simulink model "Sim_Ex36_Quiz"  (R2017a)
settings: Solver=VariableStepAuto  StartTime=0.0  StopTime=Stop_Time  MaxStep=Ts  RelTol=1e-3
values from neighbouring files (symbols this model uses):
  Cdc = 3.3e-3    (= 0.0033)    [A_Ex36.m]
  Ls = 2e-3    (= 0.002)    [A_Ex36.m]
  Ls_Hat = 1.0*Ls    (= 0.002)    [A_Ex36.m]
  Pload = 0    [A_Ex36.m]
  Rs = 0.1    [A_Ex36.m]
  Time_Pload = 0.1    [A_Ex36.m]
  Time_Vdc_Ref = 0.1    [A_Ex36.m]
  Ts = 1/fs    (= 5e-05)    [A_Ex36.m]
  Tsw = 1/fsw    (= 0.0001)    [A_Ex36.m]
  Vdc_Init = 450    [A_Ex36.m]
  Vdc_Ref = Vdc_OP    (= 500)    [A_Ex36.m]
undefined symbols (not defined in the file or in its folder): CC, DiscIntNeverNeededParam, Grid, Mode, NF, PLL, VC
libraries: simulink x2
settings Model: SimulationMode=accelerator  Creator=Joonhee  LastModifiedBy=Joonhee
settings SolverCC: MaxConsecutiveMinStep=1000

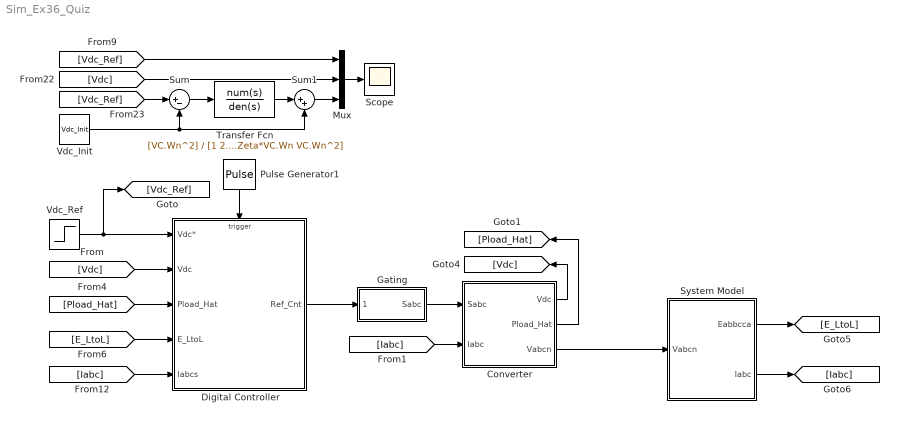
== system Sim_Ex36_Quiz ==
  Converter : Subsystem
  Digital Controller : Subsystem
  Gating : Subsystem
  Mux : Mux  Inputs=3
  Pulse Generator1 : DiscretePulseGenerator  PulseType=Time based  Period=Ts  PulseWidth=50
  Scope : Scope
  Sum : Sum  Inputs=|+-
  Sum1 : Sum  Inputs=|++
  System Model : Subsystem
  Transfer Fcn : TransferFcn  Numerator=[VC.Wn^2]  Denominator=[1 2*VC.Zeta*VC.Wn VC.Wn^2]
  Vdc_Init : Constant  Value=Vdc_Init
  Vdc_Ref : Step  Time=Time_Vdc_Ref  Before=Vdc_Init  After=Vdc_Ref  SampleTime=0
  wires:
  System Model/2(Iabc) -> [Iabc]
  [E_LtoL] -> Digital Controller/4(E_LtoL)
  Gating/1(Sabc) -> Converter/1(Sabc)
  System Model/1(Eabbcca) -> [E_LtoL]
  [Iabc] -> Converter/2(Iabc)
  [Iabc] -> Digital Controller/5(Iabcs)
  Pulse Generator1/1 -> Digital Controller/Trigger
  Converter/3(Vabcn) -> System Model/1(Vabcn)
  Digital Controller/1(Ref_Cnt) -> Gating/1(Ref_Cnt)
  Converter/1(Vdc) -> [Vdc]
  [Vdc] -> Digital Controller/2(Vdc)
  Vdc_Ref/1 -> [Vdc_Ref], Digital Controller/1(Vdc*)
  Converter/2(Pload_Hat) -> [Pload_Hat]
  [Pload_Hat] -> Digital Controller/3(Pload_Hat)
  [Vdc] -> Mux/2
  Sum1/1 -> Mux/3
  Mux/1 -> Scope/1
  Sum/1 -> Transfer Fcn/1
  [Vdc_Ref] -> Mux/1
  Vdc_Init/1 -> Sum1/2, Sum/2
  Transfer Fcn/1 -> Sum1/1
  [Vdc_Ref] -> Sum/1

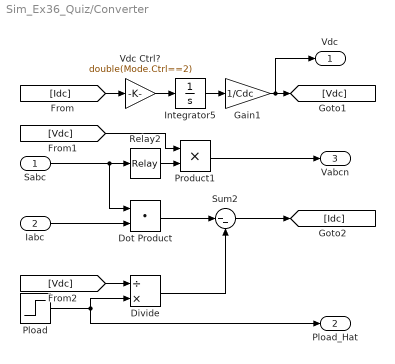
== system Sim_Ex36_Quiz/Converter ==
  Sabc : Inport
  Iabc : Inport  Port=2
  Divide : Product  Inputs=/*
  Dot Product : DotProduct  InputSameDT=on  OutDataTypeStr=Inherit: Inherit via internal rule
  Gain1 : Gain  Gain=1/Cdc
  Integrator5 : Integrator  InitialCondition=Cdc*Vdc_Init  LowerSaturationLimit=0
  Pload : Step  Time=Time_Pload  After=Pload  SampleTime=0
  Product1 : Product  RndMeth=Zero
  Relay2 : Relay  OnSwitchValue=0.5  OffSwitchValue=0.5  OnOutputValue=1/2  OffOutputValue=-1/2  OutDataTypeStr=double
  Sum2 : Sum  Inputs=|--
  Vdc Ctrl? : Gain  Gain=double(Mode.Ctrl==2)
  Vdc : Outport
  Pload_Hat : Outport  Port=2
  Vabcn : Outport  Port=3
  wires:
  [Vdc] -> Product1/1
  Sabc/1 -> Dot Product/1, Relay2/1
  Relay2/1 -> Product1/2
  Iabc/1 -> Dot Product/2
  Dot Product/1 -> Sum2/1
  Divide/1 -> Sum2/2
  Sum2/1 -> [Idc]
  Vdc Ctrl?/1 -> Integrator5/1
  Integrator5/1 -> Gain1/1
  Gain1/1 -> Vdc/1, [Vdc]
  [Idc] -> Vdc Ctrl?/1
  Product1/1 -> Vabcn/1
  [Vdc] -> Divide/1
  Pload/1 -> Pload_Hat/1, Divide/2

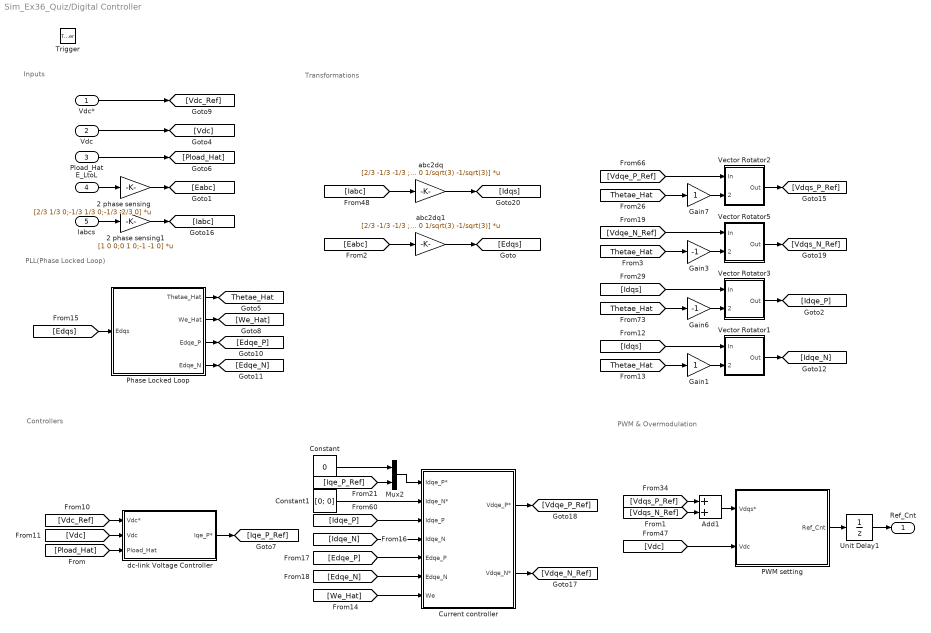
== system Sim_Ex36_Quiz/Digital Controller ==
  note: Controllers
  note: PLL(Phase Locked Loop)
  note: Inputs
  note: Transformations
  note: PWM & Overmodulation
  Vdc* : Inport
  Vdc : Inport  Port=2
  Pload_Hat : Inport  Port=3
  E_LtoL : Inport  Port=4
  Iabcs : Inport  Port=5
  Trigger : TriggerPort  VariantControl=Variant
  2 phase sensing : Gain  Gain=[2/3 1/3 0;-1/3 1/3 0;-1/3 -2/3 0]  Multiplication=Matrix(K*u)  SaturateOnIntegerOverflow=on  OutDataTypeStr=Inherit: Same as input  ParamDataTypeStr=Inherit: Same as input
  2 phase sensing1 : Gain  Gain=[1 0 0;0 1 0;-1 -1 0]  Multiplication=Matrix(K*u)  SaturateOnIntegerOverflow=on  OutDataTypeStr=Inherit: Same as input  ParamDataTypeStr=Inherit: Same as input
  Add1 : Sum
  Constant : Constant  Value=0
  Constant1 : Constant  Value=[0; 0]
  Current controller : Subsystem
  Gain1 : Gain
  Gain3 : Gain  Gain=-1
  Gain6 : Gain  Gain=-1
  Gain7 : Gain
  Mux2 : Mux  Inputs=2
  PWM setting : Subsystem
  Phase Locked Loop : Subsystem
  Unit Delay1 : UnitDelay  SampleTime=-1
  Vector Rotator1 : Subsystem
  Vector Rotator2 : Subsystem
  Vector Rotator3 : Subsystem
  Vector Rotator5 : Subsystem
  abc2dq : Gain  Gain=[2/3 -1/3 -1/3 ; 0 1/sqrt(3) -1/sqrt(3)]  Multiplication=Matrix(K*u)  SaturateOnIntegerOverflow=on  OutDataTypeStr=Inherit: Same as input  ParamDataTypeStr=Inherit: Same as input
  abc2dq1 : Gain  Gain=[2/3 -1/3 -1/3 ; 0 1/sqrt(3) -1/sqrt(3)]  Multiplication=Matrix(K*u)  SaturateOnIntegerOverflow=on  OutDataTypeStr=Inherit: Same as input  ParamDataTypeStr=Inherit: Same as input
  dc-link Voltage Controller : Subsystem
  Ref_Cnt : Outport  InitialOutput=[0]
  tag scope: Thetae_Hat=global
  wires:
  [Idqe_P] -> Current controller/3(Idqe_P)
  abc2dq/1 -> [Idqs]
  [Iabc] -> abc2dq/1
  [We_Hat] -> Current controller/7(We)
  Unit Delay1/1 -> Ref_Cnt/1
  [Thetae_Hat] -> Gain7/1
  Gain7/1 -> Vector Rotator2/2(Theta)
  [Vdqe_P_Ref] -> Vector Rotator2/1(In)
  Vector Rotator2/1(Out) -> [Vdqs_P_Ref]
  Gain6/1 -> Vector Rotator3/2(Theta)
  [Idqs] -> Vector Rotator3/1(In)
  Vector Rotator3/1(Out) -> [Idqe_P]
  [Thetae_Hat] -> Gain6/1
  Iabcs/1 -> 2 phase sensing1/1
  2 phase sensing1/1 -> [Iabc]
  [Edqs] -> Phase Locked Loop/1(Edqs)
  2 phase sensing/1 -> [Eabc]
  E_LtoL/1 -> 2 phase sensing/1
  [Eabc] -> abc2dq1/1
  abc2dq1/1 -> [Edqs]
  Phase Locked Loop/2(We_Hat) -> [We_Hat]
  [Edqe_P] -> Current controller/5(Edqe_P)
  [Edqe_N] -> Current controller/6(Edqe_N)
  [Thetae_Hat] -> Gain1/1
  Vector Rotator1/1(Out) -> [Idqe_N]
  Gain1/1 -> Vector Rotator1/2(Theta)
  [Idqs] -> Vector Rotator1/1(In)
  Current controller/2(Vdqe_N*) -> [Vdqe_N_Ref]
  [Idqe_N] -> Current controller/4(Idqe_N)
  Vector Rotator5/1(Out) -> [Vdqs_N_Ref]
  [Vdqe_N_Ref] -> Vector Rotator5/1(In)
  Gain3/1 -> Vector Rotator5/2(Theta)
  [Thetae_Hat] -> Gain3/1
  Phase Locked Loop/3(Edqe_P) -> [Edqe_P]
  Phase Locked Loop/4(Edqe_N) -> [Edqe_N]
  Phase Locked Loop/1(Thetae_Hat) -> [Thetae_Hat]
  Current controller/1(Vdqe_P*) -> [Vdqe_P_Ref]
  Vdc/1 -> [Vdc]
  dc-link Voltage Controller/1(Iqe_P*) -> [Iqe_P_Ref]
  [Vdc] -> dc-link Voltage Controller/2(Vdc)
  [Vdc_Ref] -> dc-link Voltage Controller/1(Vdc*)
  Vdc*/1 -> [Vdc_Ref]
  [Iqe_P_Ref] -> Mux2/2
  Mux2/1 -> Current controller/1(Idqe_P*)
  Constant/1 -> Mux2/1
  Pload_Hat/1 -> [Pload_Hat]
  [Pload_Hat] -> dc-link Voltage Controller/3(Pload_Hat)
  [Vdc] -> PWM setting/2(Vdc)
  [Vdqs_P_Ref] -> Add1/1
  [Vdqs_N_Ref] -> Add1/2
  PWM setting/1(Ref_Cnt) -> Unit Delay1/1
  Add1/1 -> PWM setting/1(Vdqs*)
  Constant1/1 -> Current controller/2(Idqe_N*)

== system Sim_Ex36_Quiz/Gating ==
  Ref_Cnt : Inport
  Add3 : Sum  Inputs=+-
  Relay3 : Relay  OnSwitchValue=10*eps  OffSwitchValue=-10*eps  OutDataTypeStr=double
  Repeating Sequence1 : simulink/Sources/Repeating Sequence  rep_seq_t=[0 Tsw/2 Tsw]  rep_seq_y=[0 1 0]
  Sabc : Outport
  wires:
  Add3/1 -> Relay3/1
  Relay3/1 -> Sabc/1
  Repeating Sequence1/1 -> Add3/2
  Ref_Cnt/1 -> Add3/1

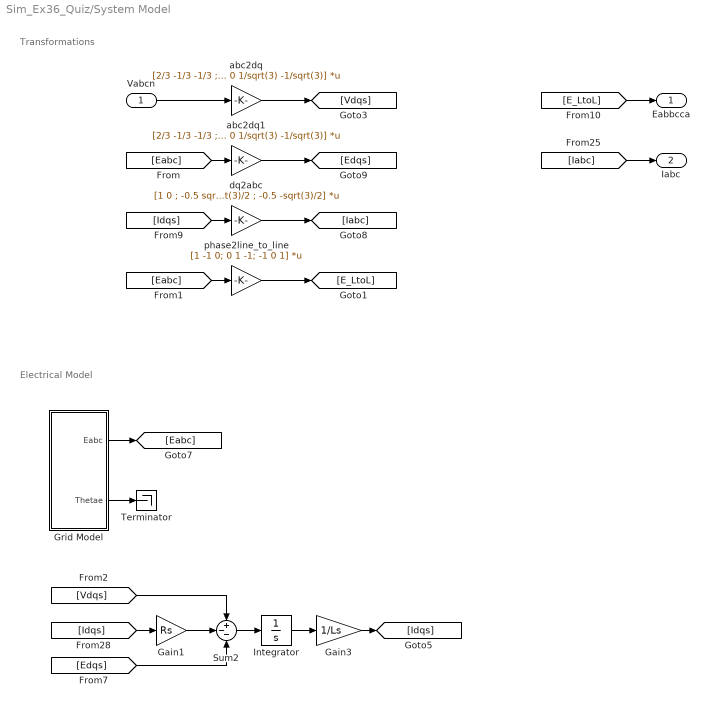
== system Sim_Ex36_Quiz/System Model ==
  note: Electrical Model
  note: Transformations
  Vabcn : Inport
  Gain1 : Gain  Gain=Rs
  Gain3 : Gain  Gain=1/Ls
  Grid Model : Subsystem
  Integrator : Integrator
  Sum2 : Sum  Inputs=+--
  Terminator : Terminator
  abc2dq : Gain  Gain=[2/3 -1/3 -1/3 ; 0 1/sqrt(3) -1/sqrt(3)]  Multiplication=Matrix(K*u)  SaturateOnIntegerOverflow=on  OutDataTypeStr=Inherit: Same as input  ParamDataTypeStr=Inherit: Same as input
  abc2dq1 : Gain  Gain=[2/3 -1/3 -1/3 ; 0 1/sqrt(3) -1/sqrt(3)]  Multiplication=Matrix(K*u)  SaturateOnIntegerOverflow=on  OutDataTypeStr=Inherit: Same as input  ParamDataTypeStr=Inherit: Same as input
  dq2abc : Gain  Gain=[1 0 ; -0.5 sqrt(3)/2 ; -0.5 -sqrt(3)/2]  Multiplication=Matrix(K*u)
  phase2line_to_line : Gain  Gain=[1 -1 0; 0 1 -1; -1 0 1]  Multiplication=Matrix(K*u)
  Eabbcca : Outport
  Iabc : Outport  Port=2
  wires:
  [Idqs] -> Gain1/1
  Vabcn/1 -> abc2dq/1
  [Idqs] -> dq2abc/1
  dq2abc/1 -> [Iabc]
  [Iabc] -> Iabc/1
  [Eabc] -> abc2dq1/1
  abc2dq1/1 -> [Edqs]
  Integrator/1 -> Gain3/1
  Gain3/1 -> [Idqs]
  Sum2/1 -> Integrator/1
  [E_LtoL] -> Eabbcca/1
  abc2dq/1 -> [Vdqs]
  [Vdqs] -> Sum2/1
  [Eabc] -> phase2line_to_line/1
  phase2line_to_line/1 -> [E_LtoL]
  Gain1/1 -> Sum2/2
  [Edqs] -> Sum2/3
  Grid Model/2(Thetae) -> Terminator/1
  Grid Model/1(Eabc) -> [Eabc]

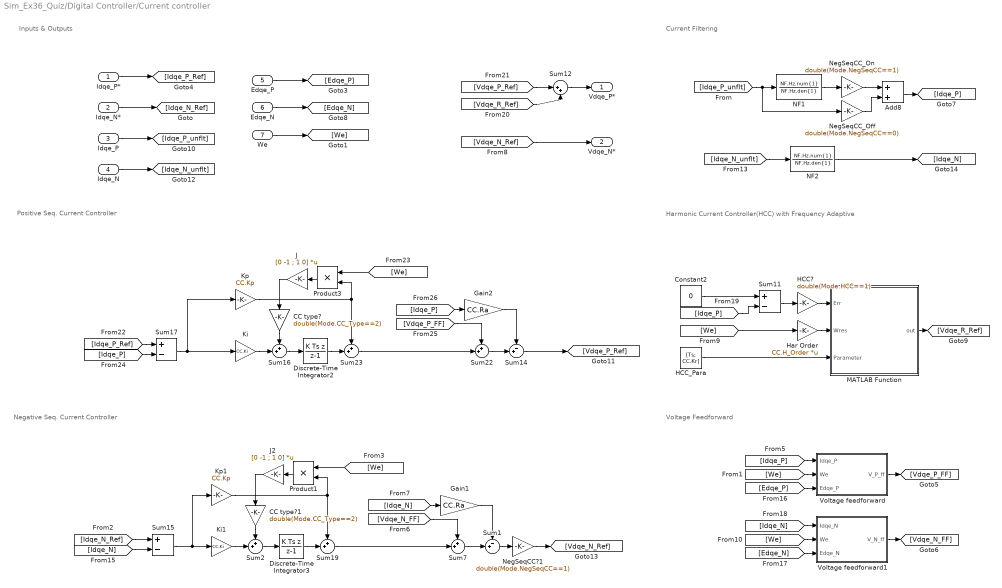
== system Sim_Ex36_Quiz/Digital Controller/Current controller ==
  note: Positive Seq. Current Controller
  note: Negative Seq. Current Controller
  note: Inputs & Outputs
  note: Voltage Feedforward
  note: Harmonic Current Controller(HCC)
      | with Frequency Adaptive
  note: Current Filtering
  Idqe_P* : Inport
  Idqe_N* : Inport  Port=2
  Idqe_P : Inport  Port=3
  Idqe_N : Inport  Port=4
  Edqe_P : Inport  Port=5
  Edqe_N : Inport  Port=6
  We : Inport  Port=7
  Add8 : Sum
  CC type? : Gain  Gain=double(Mode.CC_Type==2)
  CC type?1 : Gain  Gain=double(Mode.CC_Type==2)
  Constant2 : Constant  Value=0
  Discrete-Time Integrator2 : DiscreteIntegrator  IntegratorMethod=Integration: Backward Euler  SampleTime=-1  ICPrevOutput=DiscIntNeverNeededParam  ICPrevScaledInput=DiscIntNeverNeededParam
  Discrete-Time Integrator3 : DiscreteIntegrator  IntegratorMethod=Integration: Backward Euler  SampleTime=-1  ICPrevOutput=DiscIntNeverNeededParam  ICPrevScaledInput=DiscIntNeverNeededParam
  Gain1 : Gain  Gain=CC.Ra
  Gain2 : Gain  Gain=CC.Ra
  HCC? : Gain  Gain=double(Mode.HCC==1)
  HCC_Para : Constant  Value=[Ts; CC.Kr]
  Har Order : Gain  Gain=CC.H_Order  Multiplication=Matrix(K*u)
  J : Gain  Gain=[0 -1 ; 1 0]  Multiplication=Matrix(K*u)
  J2 : Gain  Gain=[0 -1 ; 1 0]  Multiplication=Matrix(K*u)
  Ki : Gain  Gain=CC.Ki  SaturateOnIntegerOverflow=on  OutDataTypeStr=Inherit: Same as input  ParamDataTypeStr=Inherit: Same as input
  Ki1 : Gain  Gain=CC.Ki  SaturateOnIntegerOverflow=on  OutDataTypeStr=Inherit: Same as input  ParamDataTypeStr=Inherit: Same as input
  Kp : Gain  Gain=CC.Kp  SaturateOnIntegerOverflow=on  OutDataTypeStr=Inherit: Same as input  ParamDataTypeStr=Inherit: Same as input
  Kp1 : Gain  Gain=CC.Kp  SaturateOnIntegerOverflow=on  OutDataTypeStr=Inherit: Same as input  ParamDataTypeStr=Inherit: Same as input
  MATLAB Function : MATLAB Function  TreatAsAtomicUnit=on
  NF1 : DiscreteFilter  Numerator=NF.Hz.num{1}  Denominator=NF.Hz.den{1}
  NF2 : DiscreteFilter  Numerator=NF.Hz.num{1}  Denominator=NF.Hz.den{1}
  NegSeqCC?1 : Gain  Gain=double(Mode.NegSeqCC==1)
  NegSeqCC_Off : Gain  Gain=double(Mode.NegSeqCC==0)
  NegSeqCC_On : Gain  Gain=double(Mode.NegSeqCC==1)
  Product1 : Product  RndMeth=Zero
  Product3 : Product  RndMeth=Zero
  Sum1 : Sum  Inputs=-+|
  Sum11 : Sum  Inputs=+-
  Sum12 : Sum  Inputs=|++
  Sum14 : Sum  Inputs=-+|
  Sum15 : Sum  Inputs=+-
  Sum{2,7,16,19,22..23} (6 alike) : Sum  Inputs=++|
  Sum17 : Sum  Inputs=+-
  Voltage feedforward : Subsystem
  Voltage feedforward1 : Subsystem
  Vdqe_P* : Outport
  Vdqe_N* : Outport  Port=2
  wires:
  Sum11/1 -> HCC?/1
  HCC_Para/1 -> MATLAB Function/3(Parameter)
  HCC?/1 -> MATLAB Function/1(Err)
  MATLAB Function/1(out) -> [Vdqe_R_Ref]
  Har Order/1 -> MATLAB Function/2(Wres)
  [Idqe_P] -> Sum11/2
  Constant2/1 -> Sum11/1
  [We] -> Har Order/1
  Voltage feedforward/1(V_P_ff) -> [Vdqe_P_FF]
  [Idqe_P] -> Voltage feedforward/1(Idqe_P)
  [Edqe_P] -> Voltage feedforward/3(Edqe_P)
  [We] -> Voltage feedforward1/2(We)
  [Edqe_N] -> Voltage feedforward1/3(Edqe_N)
  Voltage feedforward1/1(V_N_ff) -> [Vdqe_N_FF]
  [Idqe_N] -> Voltage feedforward1/1(Idqe_N)
  [We] -> Voltage feedforward/2(We)
  Discrete-Time Integrator2/1 -> Sum23/2
  Kp/1 -> Product3/2, Sum23/1
  Sum16/1 -> Discrete-Time Integrator2/1
  Sum14/1 -> [Vdqe_P_Ref]
  Gain2/1 -> Sum14/1
  Sum17/1 -> Ki/1, Kp/1
  [Idqe_P] -> Sum17/2
  CC type?/1 -> Sum16/1
  [Vdqe_P_FF] -> Sum22/1
  Ki/1 -> Sum16/2
  J/1 -> CC type?/1
  Sum23/1 -> Sum22/2
  [Idqe_P] -> Gain2/1
  [We] -> Product3/1
  [Idqe_P_Ref] -> Sum17/1
  Sum22/1 -> Sum14/2
  Product3/1 -> J/1
  Discrete-Time Integrator3/1 -> Sum19/2
  Sum19/1 -> Sum7/2
  [Idqe_N_Ref] -> Sum15/1
  Kp1/1 -> Product1/2, Sum19/1
  CC type?1/1 -> Sum2/1
  [Idqe_N] -> Sum15/2
  NegSeqCC?1/1 -> [Vdqe_N_Ref]
  Sum7/1 -> Sum1/2
  Sum1/1 -> NegSeqCC?1/1
  Sum15/1 -> Ki1/1, Kp1/1
  [Idqe_N] -> Gain1/1
  [We] -> Product1/1
  Ki1/1 -> Sum2/2
  [Vdqe_N_FF] -> Sum7/1
  Gain1/1 -> Sum1/1
  Sum2/1 -> Discrete-Time Integrator3/1
  Product1/1 -> J2/1
  J2/1 -> CC type?1/1
  Idqe_N*/1 -> [Idqe_N_Ref]
  [Vdqe_R_Ref] -> Sum12/2
  Idqe_P/1 -> [Idqe_P_unflt]
  Sum12/1 -> Vdqe_P*/1
  [Vdqe_P_Ref] -> Sum12/1
  Edqe_P/1 -> [Edqe_P]
  [Vdqe_N_Ref] -> Vdqe_N*/1
  Edqe_N/1 -> [Edqe_N]
  Idqe_N/1 -> [Idqe_N_unflt]
  Idqe_P*/1 -> [Idqe_P_Ref]
  We/1 -> [We]
  [Idqe_N_unflt] -> NF2/1
  NF2/1 -> [Idqe_N]
  NegSeqCC_On/1 -> Add8/1
  [Idqe_P_unflt] -> NegSeqCC_Off/1, NF1/1
  Add8/1 -> [Idqe_P]
  NF1/1 -> NegSeqCC_On/1
  NegSeqCC_Off/1 -> Add8/2

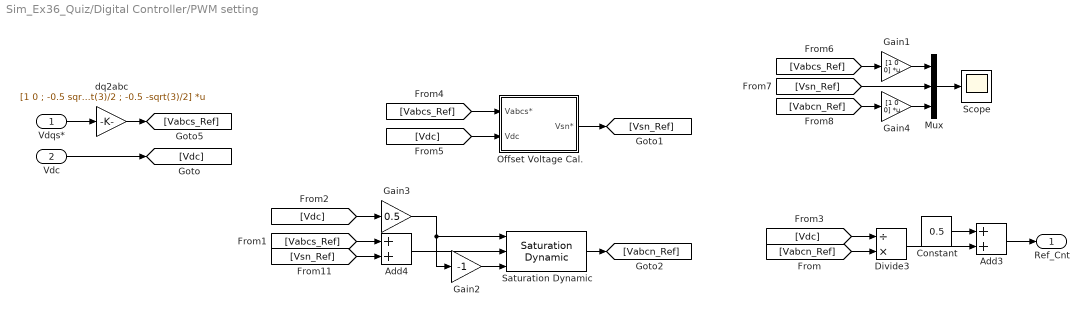
== system Sim_Ex36_Quiz/Digital Controller/PWM setting ==
  Vdqs* : Inport
  Vdc : Inport  Port=2
  Add3 : Sum
  Add4 : Sum
  Constant : Constant  Value=0.5
  Divide3 : Product  Inputs=/*
  Gain1 : Gain  Gain=[1 0 0]  Multiplication=Matrix(K*u)
  Gain2 : Gain  Gain=-1
  Gain3 : Gain  Gain=0.5
  Gain4 : Gain  Gain=[1 0 0]  Multiplication=Matrix(K*u)
  Mux : Mux  Inputs=3
  Offset Voltage Cal. : Subsystem
  Saturation Dynamic : simulink/Discontinuities/Saturation Dynamic  OutMin=[]  OutMax=[]  OutDataTypeStr=Inherit: Same as second input  OutDataType=fixdt(1, 16)  OutScaling=2^-10  DoSatur=off
  Scope : Scope
  dq2abc : Gain  Gain=[1 0 ; -0.5 sqrt(3)/2 ; -0.5 -sqrt(3)/2]  Multiplication=Matrix(K*u)
  Ref_Cnt : Outport
  wires:
  [Vdc] -> Divide3/1
  Divide3/1 -> Add3/2
  Add3/1 -> Ref_Cnt/1
  Constant/1 -> Add3/1
  Vdqs*/1 -> dq2abc/1
  Vdc/1 -> [Vdc]
  [Vdc] -> Gain3/1
  [Vabcs_Ref] -> Add4/1
  [Vsn_Ref] -> Add4/2
  Gain3/1 -> Saturation Dynamic/1, Gain2/1
  Gain2/1 -> Saturation Dynamic/3
  Add4/1 -> Saturation Dynamic/2
  dq2abc/1 -> [Vabcs_Ref]
  [Vdc] -> Offset Voltage Cal./2(Vdc)
  Offset Voltage Cal./1(Vsn*) -> [Vsn_Ref]
  [Vabcs_Ref] -> Offset Voltage Cal./1(Vabcs*)
  Saturation Dynamic/1 -> [Vabcn_Ref]
  [Vabcn_Ref] -> Divide3/2
  [Vsn_Ref] -> Mux/2
  Gain4/1 -> Mux/3
  [Vabcn_Ref] -> Gain4/1
  Gain1/1 -> Mux/1
  [Vabcs_Ref] -> Gain1/1
  Mux/1 -> Scope/1

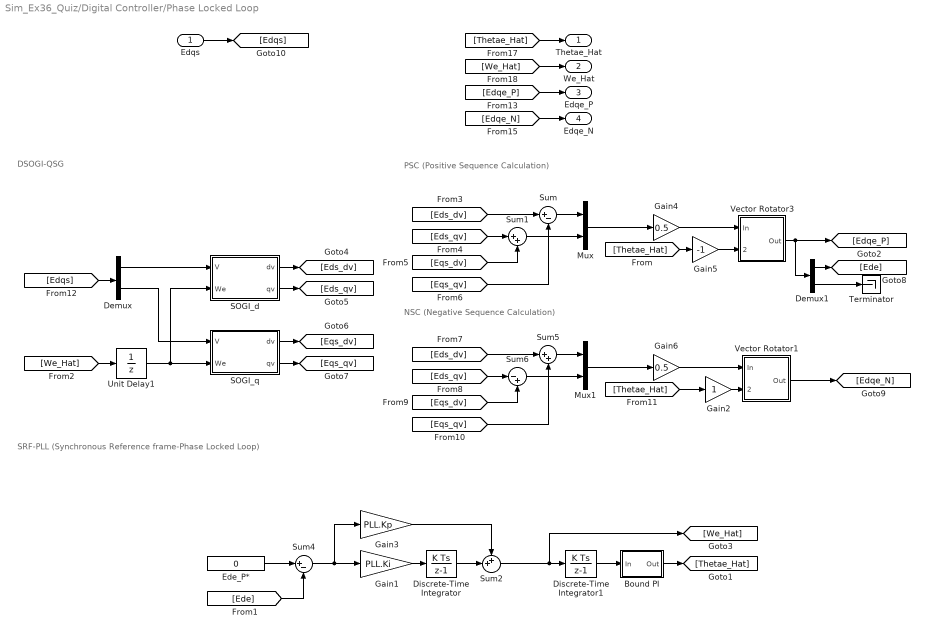
== system Sim_Ex36_Quiz/Digital Controller/Phase Locked Loop ==
  note: SRF-PLL (Synchronous Reference frame-Phase Locked Loop)
  note: PSC (Positive Sequence Calculation)
  note: DSOGI-QSG
  note: NSC (Negative Sequence Calculation)
  Edqs : Inport
  Bound PI : Subsystem
  Demux : Demux  Outputs=2
  Demux1 : Demux  Outputs=2
  Discrete-Time Integrator : DiscreteIntegrator  InitialCondition=PLL.We_FF  SampleTime=-1  ICPrevOutput=DiscIntNeverNeededParam  ICPrevScaledInput=DiscIntNeverNeededParam
  Discrete-Time Integrator1 : DiscreteIntegrator  InitialCondition=Grid.Thetae_Init  SampleTime=-1  ICPrevOutput=DiscIntNeverNeededParam  ICPrevScaledInput=DiscIntNeverNeededParam
  Ede_P* : Constant  Value=0
  Gain1 : Gain  Gain=PLL.Ki
  Gain2 : Gain
  Gain3 : Gain  Gain=PLL.Kp
  Gain4 : Gain  Gain=0.5
  Gain5 : Gain  Gain=-1
  Gain6 : Gain  Gain=0.5
  Mux : Mux  Inputs=2
  Mux1 : Mux  Inputs=2
  SOGI_d : Subsystem
  SOGI_q : Subsystem
  Sum : Sum  Inputs=|+-
  Sum1 : Sum  Inputs=|++
  Sum2 : Sum  Inputs=++|
  Sum4 : Sum  Inputs=|+-
  Sum5 : Sum  Inputs=|++
  Sum6 : Sum  Inputs=|-+
  Terminator : Terminator
  Unit Delay1 : UnitDelay  SampleTime=-1
  Vector Rotator1 : Subsystem  Tag=dqs2dqw
  Vector Rotator3 : Subsystem  Tag=dqs2dqw
  Thetae_Hat : Outport
  We_Hat : Outport  Port=2
  Edqe_P : Outport  Port=3
  Edqe_N : Outport  Port=4
  wires:
  [Edqs] -> Demux/1
  Demux/1 -> SOGI_d/1(V)
  Demux/2 -> SOGI_q/1(V)
  Ede_P*/1 -> Sum4/1
  [Ede] -> Sum4/2
  Sum4/1 -> Gain3/1, Gain1/1
  Gain1/1 -> Discrete-Time Integrator/1
  [We_Hat] -> Unit Delay1/1
  Mux/1 -> Gain4/1
  SOGI_d/1(dv) -> [Eds_dv]
  SOGI_d/2(qv) -> [Eds_qv]
  SOGI_q/1(dv) -> [Eqs_dv]
  SOGI_q/2(qv) -> [Eqs_qv]
  [Eqs_dv] -> Sum1/2
  Sum/1 -> Mux/1
  [Eqs_qv] -> Sum/2
  Sum1/1 -> Mux/2
  [Eds_dv] -> Sum/1
  [Eds_qv] -> Sum1/1
  Edqs/1 -> [Edqs]
  [We_Hat] -> We_Hat/1
  [Thetae_Hat] -> Thetae_Hat/1
  [Edqe_P] -> Edqe_P/1
  [Edqe_N] -> Edqe_N/1
  Vector Rotator3/1(Out) -> Demux1/1, [Edqe_P]
  Demux1/2 -> Terminator/1
  Demux1/1 -> [Ede]
  Gain4/1 -> Vector Rotator3/1(In)
  Unit Delay1/1 -> SOGI_q/2(We), SOGI_d/2(We)
  Sum2/1 -> [We_Hat], Discrete-Time Integrator1/1
  [Thetae_Hat] -> Gain5/1
  Discrete-Time Integrator/1 -> Sum2/2
  Gain3/1 -> Sum2/1
  Mux1/1 -> Gain6/1
  Sum6/1 -> Mux1/2
  [Eqs_qv] -> Sum5/2
  [Eqs_dv] -> Sum6/2
  [Thetae_Hat] -> Gain2/1
  [Eds_qv] -> Sum6/1
  Sum5/1 -> Mux1/1
  [Eds_dv] -> Sum5/1
  Gain2/1 -> Vector Rotator1/2(Theta)
  Gain6/1 -> Vector Rotator1/1(In)
  Vector Rotator1/1(Out) -> [Edqe_N]
  Bound PI/1(Out) -> [Thetae_Hat]
  Discrete-Time Integrator1/1 -> Bound PI/1(In)
  Gain5/1 -> Vector Rotator3/2(Theta)

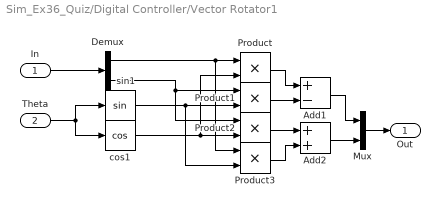
== system Sim_Ex36_Quiz/Digital Controller/Vector Rotator1 ==
  In : Inport
  Theta : Inport  Port=2
  Add1 : Sum  Inputs=+-
  Add2 : Sum
  Demux : Demux  Outputs=2
  Mux : Mux  Inputs=[1 1]
  Product{,1..3} (4 alike) : Product  RndMeth=Zero
  cos1 : Trigonometry  Operator=cos
  sin1 : Trigonometry
  Out : Outport
  wires:
  Add2/1 -> Mux/2
  Product3/1 -> Add2/2
  Product2/1 -> Add2/1
  Add1/1 -> Mux/1
  Product1/1 -> Add1/2
  Product/1 -> Add1/1
  sin1/1 -> Product3/2, Product1/2
  cos1/1 -> Product2/2, Product/2
  Demux/2 -> Product2/1, Product1/1
  In/1 -> Demux/1
  Mux/1 -> Out/1
  Demux/1 -> Product/1, Product3/1
  Theta/1 -> sin1/1, cos1/1

== system Sim_Ex36_Quiz/Digital Controller/Vector Rotator2 ==
  In : Inport
  Theta : Inport  Port=2
  Add1 : Sum  Inputs=+-
  Add2 : Sum
  Demux : Demux  Outputs=2
  Mux : Mux  Inputs=[1 1]
  Product{,1..3} (4 alike) : Product  RndMeth=Zero
  cos1 : Trigonometry  Operator=cos
  sin1 : Trigonometry
  Out : Outport
  wires:
  Theta/1 -> cos1/1, sin1/1
  Demux/1 -> Product3/1, Product/1
  Mux/1 -> Out/1
  In/1 -> Demux/1
  Demux/2 -> Product1/1, Product2/1
  cos1/1 -> Product/2, Product2/2
  sin1/1 -> Product1/2, Product3/2
  Product/1 -> Add1/1
  Product1/1 -> Add1/2
  Add1/1 -> Mux/1
  Product2/1 -> Add2/1
  Product3/1 -> Add2/2
  Add2/1 -> Mux/2

== system Sim_Ex36_Quiz/Digital Controller/Vector Rotator3 ==
  In : Inport
  Theta : Inport  Port=2
  Add1 : Sum  Inputs=+-
  Add2 : Sum
  Demux : Demux  Outputs=2
  Mux : Mux  Inputs=[1 1]
  Product{,1..3} (4 alike) : Product  RndMeth=Zero
  cos1 : Trigonometry  Operator=cos
  sin1 : Trigonometry
  Out : Outport
  wires:
  Theta/1 -> cos1/1, sin1/1
  Demux/1 -> Product3/1, Product/1
  Mux/1 -> Out/1
  In/1 -> Demux/1
  Demux/2 -> Product1/1, Product2/1
  cos1/1 -> Product/2, Product2/2
  sin1/1 -> Product1/2, Product3/2
  Product/1 -> Add1/1
  Product1/1 -> Add1/2
  Add1/1 -> Mux/1
  Product2/1 -> Add2/1
  Product3/1 -> Add2/2
  Add2/1 -> Mux/2

== system Sim_Ex36_Quiz/Digital Controller/Vector Rotator5 ==
  In : Inport
  Theta : Inport  Port=2
  Add1 : Sum  Inputs=+-
  Add2 : Sum
  Demux : Demux  Outputs=2
  Mux : Mux  Inputs=[1 1]
  Product{,1..3} (4 alike) : Product  RndMeth=Zero
  cos1 : Trigonometry  Operator=cos
  sin1 : Trigonometry
  Out : Outport
  wires:
  Add2/1 -> Mux/2
  Product3/1 -> Add2/2
  Product2/1 -> Add2/1
  Add1/1 -> Mux/1
  Product1/1 -> Add1/2
  Product/1 -> Add1/1
  sin1/1 -> Product3/2, Product1/2
  cos1/1 -> Product2/2, Product/2
  Demux/2 -> Product2/1, Product1/1
  In/1 -> Demux/1
  Mux/1 -> Out/1
  Demux/1 -> Product/1, Product3/1
  Theta/1 -> sin1/1, cos1/1

== system Sim_Ex36_Quiz/Digital Controller/dc-link Voltage Controller ==
  Vdc* : Inport
  Vdc : Inport  Port=2
  Pload_Hat : Inport  Port=3
  Discrete-Time Integrator : DiscreteIntegrator  IntegratorMethod=Integration: Backward Euler  InitialCondition=VC.Kp*Vdc_Init  SampleTime=-1  ICPrevOutput=DiscIntNeverNeededParam  ICPrevScaledInput=DiscIntNeverNeededParam
  Gain : Gain  Gain=-1
  Gain1 : Gain  Gain=1/(1.5*E)
  Gain17 : Gain  Gain=VC.Ki
  Gain3 : Gain  Gain=VC.Kp
  Sum : Sum  Inputs=-+|
  Sum1 : Sum  Inputs=|+-
  Sum2 : Sum  Inputs=-+|
  Sum3 : Sum  Inputs=++|
  Iqe_P* : Outport  InitialOutput=[0]

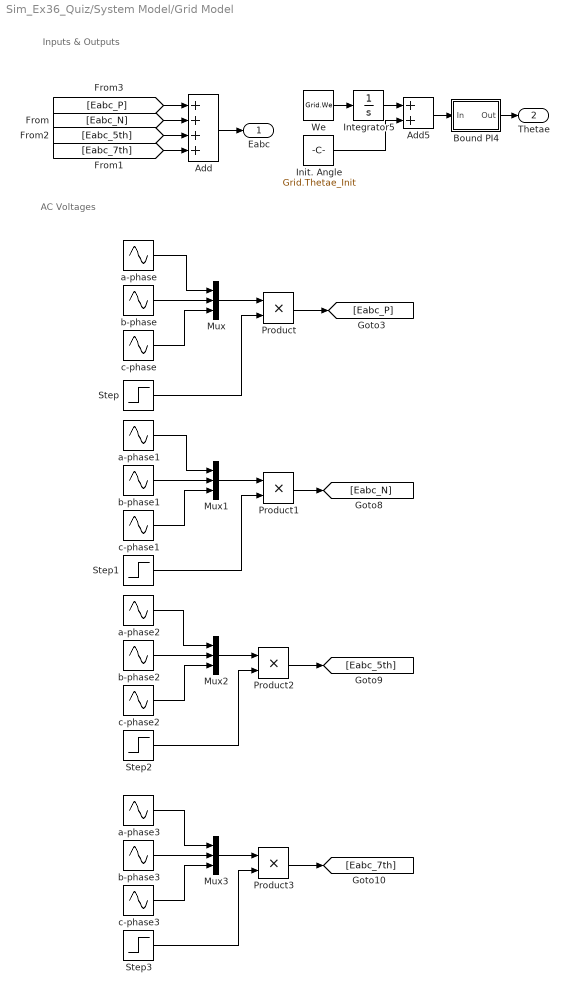
== system Sim_Ex36_Quiz/System Model/Grid Model ==
  note: AC Voltages
  note: Inputs & Outputs
  Add : Sum  Inputs=++++
  Add5 : Sum
  Bound PI4 : Subsystem
  Init. Angle : Constant  Value=Grid.Thetae_Init
  Integrator5 : Integrator
  Mux{,1..3} (4 alike) : Mux  Inputs=3
  Product{,1..3} (4 alike) : Product
  Step : Step  Time=Grid.Time_Fault  Before=1  After=Grid.Ratio_P  SampleTime=0
  Step1 : Step  Time=Grid.Time_Fault  SampleTime=0
  Step2 : Step  Time=Grid.Time_Fault  SampleTime=0
  Step3 : Step  Time=Grid.Time_Fault  SampleTime=0
  We : Constant  Value=Grid.We
  a-phase : Sin  Amplitude=Grid.V_P  Frequency=Grid.We  Phase=Grid.Thetae_Init+pi  SampleTime=0
  a-phase1 : Sin  Amplitude=Grid.V_N  Frequency=Grid.We  Phase=Grid.Thetae_N_Init+pi  SampleTime=0
  a-phase2 : Sin  Amplitude=Grid.V_5th  Frequency=5*Grid.We  Phase=Grid.Thetae_5th_Init+pi  SampleTime=0
  a-phase3 : Sin  Amplitude=Grid.V_7th  Frequency=7*Grid.We  Phase=Grid.Thetae_7th_Init+pi  SampleTime=0
  b-phase : Sin  Amplitude=Grid.V_P  Frequency=Grid.We  Phase=Grid.Thetae_Init+pi-2/3*pi  SampleTime=0
  b-phase1 : Sin  Amplitude=Grid.V_N  Frequency=Grid.We  Phase=Grid.Thetae_N_Init+pi+2/3*pi  SampleTime=0
  b-phase2 : Sin  Amplitude=Grid.V_5th  Frequency=5*Grid.We  Phase=Grid.Thetae_5th_Init+pi+2/3*pi  SampleTime=0
  b-phase3 : Sin  Amplitude=Grid.V_7th  Frequency=7*Grid.We  Phase=Grid.Thetae_7th_Init+pi-2/3*pi  SampleTime=0
  c-phase : Sin  Amplitude=Grid.V_P  Frequency=Grid.We  Phase=Grid.Thetae_Init+pi-4/3*pi  SampleTime=0
  c-phase1 : Sin  Amplitude=Grid.V_N  Frequency=Grid.We  Phase=Grid.Thetae_N_Init+pi+4/3*pi  SampleTime=0
  c-phase2 : Sin  Amplitude=Grid.V_5th  Frequency=5*Grid.We  Phase=Grid.Thetae_5th_Init+pi+4/3*pi  SampleTime=0
  c-phase3 : Sin  Amplitude=Grid.V_7th  Frequency=7*Grid.We  Phase=Grid.Thetae_7th_Init+pi-4/3*pi  SampleTime=0
  Eabc : Outport
  Thetae : Outport  Port=2
  wires:
  [Eabc_P] -> Add/1
  Add/1 -> Eabc/1
  [Eabc_N] -> Add/2
  [Eabc_5th] -> Add/3
  [Eabc_7th] -> Add/4
  Bound PI4/1(Out) -> Thetae/1
  Add5/1 -> Bound PI4/1(In)
  We/1 -> Integrator5/1
  Init. Angle/1 -> Add5/2
  Integrator5/1 -> Add5/1
  b-phase/1 -> Mux/2
  a-phase/1 -> Mux/1
  c-phase/1 -> Mux/3
  c-phase1/1 -> Mux1/3
  a-phase1/1 -> Mux1/1
  b-phase1/1 -> Mux1/2
  b-phase2/1 -> Mux2/2
  a-phase2/1 -> Mux2/1
  c-phase2/1 -> Mux2/3
  c-phase3/1 -> Mux3/3
  a-phase3/1 -> Mux3/1
  b-phase3/1 -> Mux3/2
  Mux/1 -> Product/1
  Mux1/1 -> Product1/1
  Step/1 -> Product/2
  Product/1 -> [Eabc_P]
  Step1/1 -> Product1/2
  Mux2/1 -> Product2/1
  Mux3/1 -> Product3/1
  Step2/1 -> Product2/2
  Step3/1 -> Product3/2
  Product1/1 -> [Eabc_N]
  Product2/1 -> [Eabc_5th]
  Product3/1 -> [Eabc_7th]

== system Sim_Ex36_Quiz/Digital Controller/Current controller/Voltage feedforward ==
  Idqe_P : Inport
  We : Inport  Port=2
  Edqe_P : Inport  Port=3
  CC type : Gain  Gain=double(Mode.CC_Type==1)
  J : Gain  Gain=[0 -1 ; 1 0]  Multiplication=Matrix(K*u)
  Ls_Hat : Gain  Gain=Ls_Hat
  Product : Product  RndMeth=Zero
  Sum2 : Sum  Inputs=|++
  V_P_ff : Outport
  wires:
  Idqe_P/1 -> Ls_Hat/1
  We/1 -> Product/2
  J/1 -> Product/1
  Ls_Hat/1 -> CC type/1
  CC type/1 -> J/1
  Sum2/1 -> V_P_ff/1
  Edqe_P/1 -> Sum2/2
  Product/1 -> Sum2/1

== system Sim_Ex36_Quiz/Digital Controller/Current controller/Voltage feedforward1 ==
  Idqe_N : Inport
  We : Inport  Port=2
  Edqe_N : Inport  Port=3
  CC type : Gain  Gain=double(Mode.CC_Type==1)
  J : Gain  Gain=[0 -1 ; 1 0]  Multiplication=Matrix(K*u)
  Ls_Hat : Gain  Gain=Ls_Hat
  Product1 : Product  RndMeth=Zero
  Sum1 : Sum  Inputs=|-+
  V_N_ff : Outport
  wires:
  Edqe_N/1 -> Sum1/2
  Idqe_N/1 -> Ls_Hat/1
  We/1 -> Product1/2
  J/1 -> Product1/1
  Ls_Hat/1 -> CC type/1
  CC type/1 -> J/1
  Product1/1 -> Sum1/1
  Sum1/1 -> V_N_ff/1

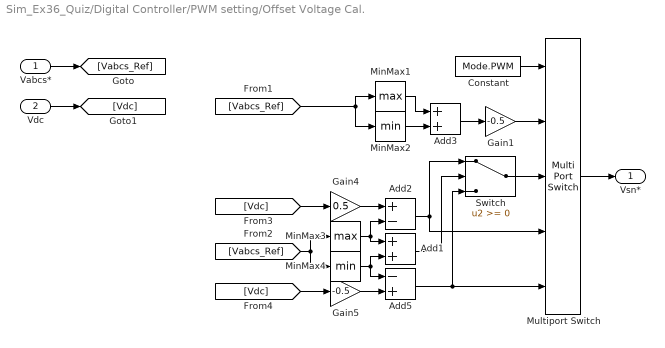
== system Sim_Ex36_Quiz/Digital Controller/PWM setting/Offset Voltage Cal. ==
  Vabcs* : Inport
  Vdc : Inport  Port=2
  Add1 : Sum
  Add2 : Sum  Inputs=+-
  Add3 : Sum
  Add5 : Sum  Inputs=-+
  Constant : Constant  Value=Mode.PWM
  Gain1 : Gain  Gain=-0.5
  Gain4 : Gain  Gain=0.5
  Gain5 : Gain  Gain=-0.5
  MinMax1 : MinMax  Function=max
  MinMax2 : MinMax
  MinMax3 : MinMax  Function=max
  MinMax4 : MinMax
  Multiport Switch : MultiPortSwitch  Inputs=4
  Switch : Switch
  Vsn* : Outport
  wires:
  Add2/1 -> Multiport Switch/4, Switch/1
  Add3/1 -> Gain1/1
  MinMax2/1 -> Add3/2
  MinMax1/1 -> Add3/1
  Constant/1 -> Multiport Switch/1
  Gain1/1 -> Multiport Switch/2
  MinMax3/1 -> Add2/2, Add1/1
  [Vabcs_Ref] -> MinMax3/1, MinMax4/1
  [Vabcs_Ref] -> MinMax2/1, MinMax1/1
  Multiport Switch/1 -> Vsn*/1
  Add1/1 -> Switch/2
  MinMax4/1 -> Add1/2, Add5/1
  Gain4/1 -> Add2/1
  Switch/1 -> Multiport Switch/3
  [Vdc] -> Gain5/1
  Gain5/1 -> Add5/2
  Add5/1 -> Switch/3, Multiport Switch/5
  [Vdc] -> Gain4/1
  Vabcs*/1 -> [Vabcs_Ref]
  Vdc/1 -> [Vdc]

== system Sim_Ex36_Quiz/Digital Controller/Phase Locked Loop/Bound PI ==
  In : Inport
  Fcn1 : Fcn  Expr=1/(2*pi)*u+0.5
  Fcn2 : Fcn  Expr=u-floor(u)
  Fcn3 : Fcn  Expr=2*pi*(u-0.5)
  Out : Outport
  wires:
  Fcn1/1 -> Fcn2/1
  Fcn2/1 -> Fcn3/1
  In/1 -> Fcn1/1
  Fcn3/1 -> Out/1

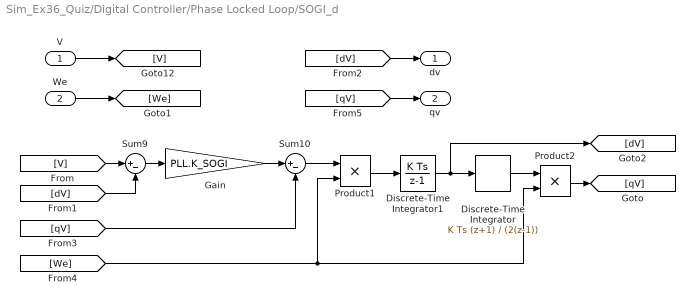
== system Sim_Ex36_Quiz/Digital Controller/Phase Locked Loop/SOGI_d ==
  V : Inport
  We : Inport  Port=2
  Discrete-Time Integrator : DiscreteIntegrator  IntegratorMethod=Integration: Trapezoidal  InitialCondition=Grid.V_P*cos(Grid.Thetae_Init+1.4*Grid.We*Ts)/PLL.We_FF  SampleTime=-1  ICPrevOutput=DiscIntNeverNeededParam  ICPrevScaledInput=DiscIntNeverNeededParam
  Discrete-Time Integrator1 : DiscreteIntegrator  InitialCondition=Grid.V_P*sin(Grid.Thetae_Init+pi+1.4*Grid.We*Ts)  SampleTime=-1  ICPrevOutput=DiscIntNeverNeededParam  ICPrevScaledInput=DiscIntNeverNeededParam
  Gain : Gain  Gain=PLL.K_SOGI
  Product1 : Product
  Product2 : Product
  Sum10 : Sum  Inputs=|+-
  Sum9 : Sum  Inputs=|+-
  dv : Outport
  qv : Outport  Port=2
  wires:
  [V] -> Sum9/1
  [dV] -> Sum9/2
  Sum9/1 -> Gain/1
  Gain/1 -> Sum10/1
  [qV] -> Sum10/2
  Sum10/1 -> Product1/1
  [We] -> Product1/2, Product2/2
  Product2/1 -> [qV]
  [dV] -> dv/1
  V/1 -> [V]
  We/1 -> [We]
  [qV] -> qv/1
  Product1/1 -> Discrete-Time Integrator1/1
  Discrete-Time Integrator1/1 -> [dV], Discrete-Time Integrator/1
  Discrete-Time Integrator/1 -> Product2/1

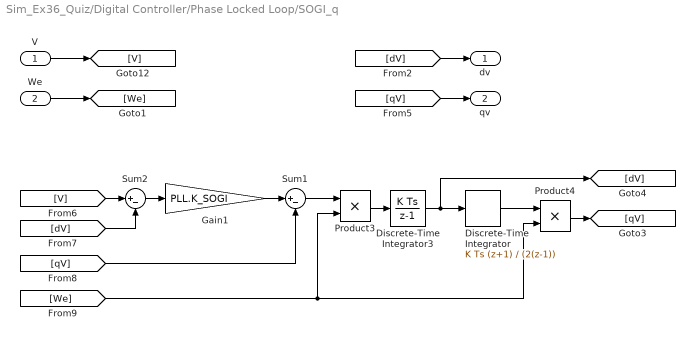
== system Sim_Ex36_Quiz/Digital Controller/Phase Locked Loop/SOGI_q ==
  V : Inport
  We : Inport  Port=2
  Discrete-Time Integrator : DiscreteIntegrator  IntegratorMethod=Integration: Trapezoidal  InitialCondition=Grid.V_P*sin(Grid.Thetae_Init+1.4*Grid.We*Ts)/PLL.We_FF  SampleTime=-1  ICPrevOutput=DiscIntNeverNeededParam  ICPrevScaledInput=DiscIntNeverNeededParam
  Discrete-Time Integrator3 : DiscreteIntegrator  InitialCondition=Grid.V_P*cos(Grid.Thetae_Init+1.4*Grid.We*Ts)  SampleTime=-1  ICPrevOutput=DiscIntNeverNeededParam  ICPrevScaledInput=DiscIntNeverNeededParam
  Gain1 : Gain  Gain=PLL.K_SOGI
  Product3 : Product
  Product4 : Product
  Sum1 : Sum  Inputs=|+-
  Sum2 : Sum  Inputs=|+-
  dv : Outport
  qv : Outport  Port=2
  wires:
  [qV] -> qv/1
  We/1 -> [We]
  V/1 -> [V]
  [dV] -> dv/1
  Product3/1 -> Discrete-Time Integrator3/1
  Product4/1 -> [qV]
  [We] -> Product3/2, Product4/2
  Gain1/1 -> Sum1/1
  [dV] -> Sum2/2
  Sum1/1 -> Product3/1
  [V] -> Sum2/1
  Sum2/1 -> Gain1/1
  Discrete-Time Integrator/1 -> Product4/1
  [qV] -> Sum1/2
  Discrete-Time Integrator3/1 -> [dV], Discrete-Time Integrator/1

== system Sim_Ex36_Quiz/Digital Controller/Phase Locked Loop/Vector Rotator1 ==
  In : Inport
  Theta : Inport  Port=2
  Add1 : Sum  Inputs=+-
  Add2 : Sum
  Demux : Demux  Outputs=2
  Mux : Mux  Inputs=[1 1]
  Product{,1..3} (4 alike) : Product  RndMeth=Zero
  cos1 : Trigonometry  Operator=cos
  sin1 : Trigonometry
  Out : Outport
  wires:
  Theta/1 -> cos1/1, sin1/1
  Demux/1 -> Product3/1, Product/1
  Mux/1 -> Out/1
  In/1 -> Demux/1
  Demux/2 -> Product1/1, Product2/1
  cos1/1 -> Product/2, Product2/2
  sin1/1 -> Product1/2, Product3/2
  Product/1 -> Add1/1
  Product1/1 -> Add1/2
  Add1/1 -> Mux/1
  Product2/1 -> Add2/1
  Product3/1 -> Add2/2
  Add2/1 -> Mux/2

== system Sim_Ex36_Quiz/Digital Controller/Phase Locked Loop/Vector Rotator3 ==
  In : Inport
  Theta : Inport  Port=2
  Add1 : Sum  Inputs=+-
  Add2 : Sum
  Demux : Demux  Outputs=2
  Mux : Mux  Inputs=[1 1]
  Product{,1..3} (4 alike) : Product  RndMeth=Zero
  cos1 : Trigonometry  Operator=cos
  sin1 : Trigonometry
  Out : Outport
  wires:
  Theta/1 -> cos1/1, sin1/1
  Demux/1 -> Product3/1, Product/1
  Mux/1 -> Out/1
  In/1 -> Demux/1
  Demux/2 -> Product1/1, Product2/1
  cos1/1 -> Product/2, Product2/2
  sin1/1 -> Product1/2, Product3/2
  Product/1 -> Add1/1
  Product1/1 -> Add1/2
  Add1/1 -> Mux/1
  Product2/1 -> Add2/1
  Product3/1 -> Add2/2
  Add2/1 -> Mux/2

== system Sim_Ex36_Quiz/System Model/Grid Model/Bound PI4 ==
  In : Inport
  Fcn1 : Fcn  Expr=1/(2*pi)*u+0.5
  Fcn2 : Fcn  Expr=u-floor(u)
  Fcn3 : Fcn  Expr=2*pi*(u-0.5)
  Out : Outport
  wires:
  Fcn1/1 -> Fcn2/1
  Fcn2/1 -> Fcn3/1
  In/1 -> Fcn1/1
  Fcn3/1 -> Out/1

== matlab function Sim_Ex36_Quiz/Digital Controller/Current controller/MATLAB Function ==
  data: Err input; out output; Wres input; Parameter input
function out = HCC(Err, Wres, Parameter)

Ts=Parameter(1);
Kr=Parameter(2);
N=length(Wres);

persistent xReg yReg

if isempty(xReg)
    xReg=zeros(2,2,N);
    yReg=zeros(2,2,N);
end
out = zeros(2,1);
a=zeros(N,1);
b=zeros(N,1);
Vres_Ref=zeros(2,N);
for i=1:N
    b(i)=2*cos(Wres(i)*Ts);
    a(i)=Kr*sin(Wres(i)*Ts)/(2*Wres(i));

    Vres_Ref(:,i)=b(i)*yReg(:,1,i)-yReg(:,2,i)+a(i)*(Err-xReg(:,2,i));
    yReg(:,2,i)=yReg(:,1,i);
    yReg(:,1,i)=Vres_Ref(:,i);

    xReg(:,2,i)=xReg(:,1,i);
    xReg(:,1,i)=Err;
    
    out = out+Vres_Ref(:,i);
end

end
